simulink model "Riggs_model"  (R2021a)
settings: Solver=VariableStepAuto  StartTime=0.0  StopTime=10.0  RelTol=1e-3
libraries: simulink x1
settings Model: Creator=SAT  LastModifiedBy=MSII

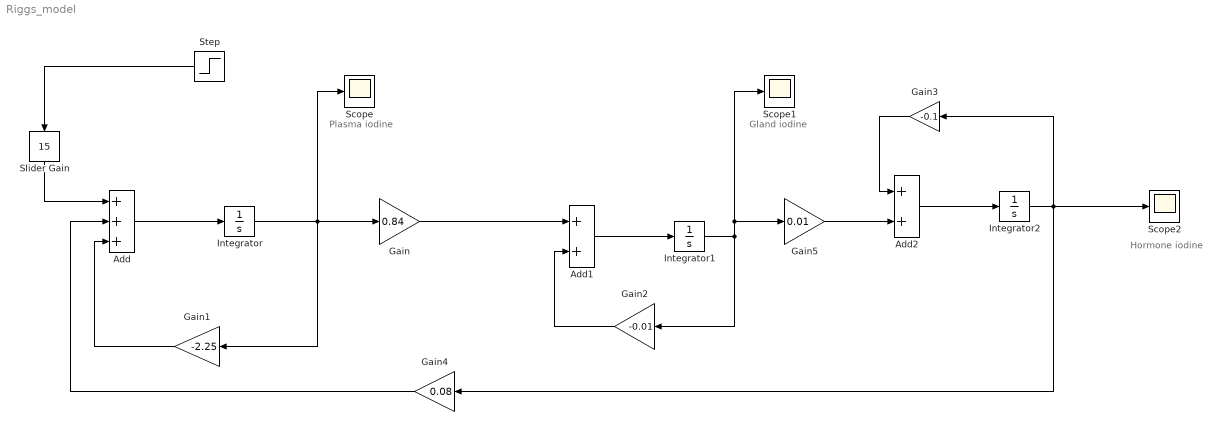
== system Riggs_model ==
  note: Plasma iodine
  note: Gland iodine
  note: Hormone iodine
  Add : Sum  Inputs=+++
  Add1 : Sum
  Add2 : Sum
  Gain : Gain  Gain=0.84
  Gain1 : Gain  Gain=-2.25
  Gain2 : Gain  Gain=-0.01
  Gain3 : Gain  Gain=-0.1
  Gain4 : Gain  Gain=0.08
  Gain5 : Gain  Gain=0.01
  Integrator : Integrator
  Integrator1 : Integrator
  Integrator2 : Integrator
  Scope : Scope
  Scope1 : Scope
  Scope2 : Scope
  Slider Gain : simulink/Math Operations/Slider Gain  gain=15  low=0  high=16
  Step : Step  Before=1  SampleTime=0
  wires:
  Step/1 -> Slider Gain/1
  Slider Gain/1 -> Add/1
  Add/1 -> Integrator/1
  Integrator/1 -> Scope/1, Gain/1, Gain1/1
  Gain/1 -> Add1/1
  Gain1/1 -> Add/3
  Add1/1 -> Integrator1/1
  Integrator1/1 -> Gain5/1, Scope1/1, Gain2/1
  Gain2/1 -> Add1/2
  Add2/1 -> Integrator2/1
  Integrator2/1 -> Gain4/1, Scope2/1, Gain3/1
  Gain3/1 -> Add2/1
  Gain4/1 -> Add/2
  Gain5/1 -> Add2/2
